simulink model "gm_cruise_control_dut_harness_mq"  (R2014b)
settings: Solver=FixedStepDiscrete  StartTime=0  StopTime=0.029999999999999999  FixedStep=0.01  RelTol=1e-3
undefined symbols (not defined in the file): sigbuilder_block
libraries: simulink x3, hdlmdlgenlib x1, modelsimlib x1
settings Model: RecordCoverage=on  CovMetricSettings=dcmoeb  covSaveCumulativeToWorkspaceVar=off  CovSaveSingleToWorkspaceVar=off  CovReportOnPause=off  CovModelRefEnable=off  CovExternalEMLEnable=on  Creator=The MathWorks Inc.  LastModifiedBy=kotsuka
settings DataIOCC: SaveFormat=StructureWithTime
settings OptimizationCC: BlockReduction=off  ConditionallyExecuteInputs=off  InlineParams=on  InlineInvariantSignals=on  ExpressionFolding=off  ExpressionDepthLimit=2147483647  InitFltsAndDblsToZero=on  EfficientMapNaN2IntZero=off
settings DebuggingCC: SaveWithParameterizedLinksMsg=none  UnderspecifiedInitializationDetection=Classic  MergeDetectMultiDrivingBlocksExec=none  SignalResolutionControl=TryResolveAllWithWarning  InheritedTsInSrcMsg=none  FcnCallInpInsideContextMsg=UseLocalSettings  StateNameClashWarn=warning
settings GRTTargetCC: TargetFcnLib=ansi_tfl_tmw.mat  CombineOutputUpdateFcns=off  GRTInterface=on
settings ConfigComp: Description=Design Verifier Custom Configuration Component  DVMaxProcessTime=60  DVMakeOutputFilesUnique=off  DVParameters=on  DVModelCoverageObjectives=MCDC  DVMaxTestCaseSteps=500  DVTestSuiteOptimization=CombinedObjectives  DVAssertions=EnableAll  DVProofAssumptions=EnableAll  DVCovFilter=on  DVDetectActiveLogic=on  DVProvingStrategy=FindViolation

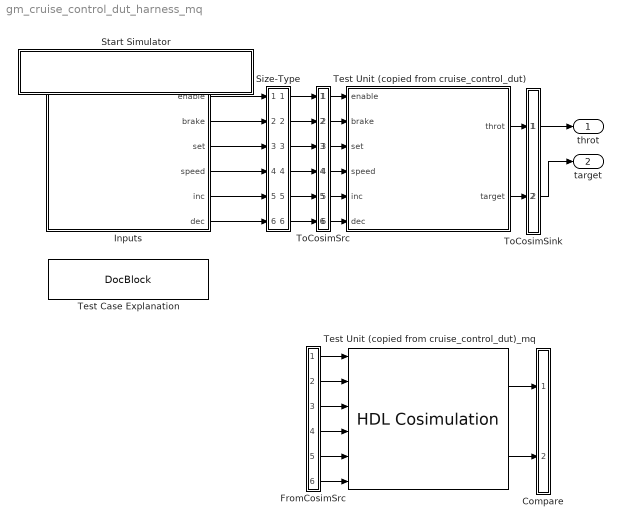
== system gm_cruise_control_dut_harness_mq ==
  Compare : Subsystem
      mask Display: disp('')
  FromCosimSrc : Subsystem
      mask Display: disp('')
  Inputs : Subsystem  Tag=STV Subsys  LoadFcn=sigbuilder_block('load');  StartFcn=sigbuilder_block('start');  StopFcn=sigbuilder_block('stop');  ClipboardFcn=sigbuilder_block('clipboard');  mask(Sigbuilder block){}
      mask init:
      | if ~strcmp(get_param(bdroot(gcb),'SimulationStatus'),'stopped'),tuvar = sigbuilder_block('maskInit'); end
      settings: CopyFcn=sigbuilder_block('copy');  DeleteFcn=sigbuilder_block('delete');  ModelCloseFcn=sigbuilder_block('modelClose');  PreSaveFcn=sigbuilder_block('preSave');  PauseFcn=sigbuilder_block('pause');  ContinueFcn=sigbuilder_block('continue');  NameChangeFcn=sigbuilder_block('namechange');  OpenFcn=sigbuilder_block('open');  CloseFcn=sigbuilder_block('close');
      mask Display: plot(0, 0, 100, 100,[2, 2, 32, 32, 2], [68, 8, 8, 68, 68],[32, 2], [38, 38], [32, 19, 2],[53, 60, 44], [32, 17, 17, 2],[16, 16, 31, 31]);txt = getActiveGroup(gcbh);text(2, 100, txt,'verticalAlignment', 'top');
  Size-Type : Subsystem
  Start Simulator : Subsystem
      settings: OpenFcn=|
      | try
      |    cosimDirName = pwd;
      |    cd 'hdlsrc\cruise_control_dut_harness';
      |    vsim('tclstart',gm_cruise_control_dut_harness_mq_tcl);
      |    cd (cosimDirName);
      |    clear cosimDirName;
      | catch me
      |    disp('Failed to launch cosimulator with "vsim"');
      |    disp (me.message);
      |    cd (cosimDirName);
      |    clear cosimDirName;
      | end
      mask Display: disp(['vsimulink -novopt work.Test_Unit_copied_from_cruise_control_dut' char(10) 'Double-click here to launch ModelSim'])
  Test Case Explanation : simulink/Model-Wide Utilities/DocBlock  DocumentType=Text
  Test Unit (copied from cruise_control_dut) : Subsystem
  Test Unit (copied from cruise_control_dut)_mq : modelsimlib/HDL Cosimulation  PortPaths=/Test_Unit_copied_from_cruise_control_dut/enable;/Test_Unit_copied_from_cruise_control_dut/brake;/Test_Unit_copied_from_cruise_control_dut/set;/Test_Unit_copied_from_cruise_control_dut/speed;/Test_Unit_copied_from_cruise_control_dut/inc;/Test_Unit_copied_from_cruise_control_dut/dec;/Test_Unit_copied_from_cruise_control_dut/throt;/Test_Unit_copied_from_cruise_control_dut/target  PortModes=[1 1 1 1 1 1 2 2 ]  PortTimes=[-1 -1 -1 -1 -1 -1 0.01 0.01 ]  PortSigns=[-1 -1 -1 -1 -1 -1 2 2 ]  PortFracLengths=[0,0,0,0,0,0,0,0]  CommLocal=on  CommSharedMemory=on  CommPortNumber=4449  CommShowInfo=on  ClockModes=[]  ClockTimes=[]  TclPreSimCommand=|  TclPostSimCommand="puts \"done\""  TimingMode=ns  TimingScaleFactor=1000  idxCellArray={'UNUSED_VAR'}  CosimBypass=Full Simulation  AllowDirectFeedthrough=on  ProductName=EDA Simulator Link MQ  RunAutoTimescale=off  HdlClocks=0  PreRunTime=40  PreRunTimeUnit=ns
      | puts "Running Simulink Cosimulation block.";
      |  puts "Chip Name: --> cruise_control_dut_harness/Test Unit (copied from cruise_control_dut)";
      |  puts "Target language: --> vhdl";
      |  puts "Target directory: --> hdlsrc\cruise_control_dut_harness";
      |  puts [clock format [clock seconds]];
      | # Clock force command;
      | force /Test_Unit_copied_from_cruise_control_dut/clk 0 0ns, 1 5ns -r 10ns;
      | # Clock enable force command;
      | force /Test_Unit_copied_from_cruise_control_dut/clk_enable 0 0ns, 1 37ns;
      | # Reset force command;
      | force /Test_Unit_copied_from_cruise_control_dut/reset 1 0ns, 0 27ns;
  ToCosimSink : Subsystem
      mask Display: disp('')
  ToCosimSrc : Subsystem
      mask Display: disp('')
  throt : Outport
  target : Outport  Port=2
  wires:
  Inputs/1(enable) -> Size-Type/1(In1)
  Inputs/2(brake) -> Size-Type/2(In2)
  Inputs/3(set) -> Size-Type/3(In3)
  Inputs/4(speed) -> Size-Type/4(In4)
  Inputs/5(inc) -> Size-Type/5(In5)
  Inputs/6(dec) -> Size-Type/6(In6)
  ToCosimSrc/1(out1) -> Test Unit (copied from cruise_control_dut)/1(enable)
  ToCosimSrc/2(out2) -> Test Unit (copied from cruise_control_dut)/2(brake)
  ToCosimSrc/3(out3) -> Test Unit (copied from cruise_control_dut)/3(set)
  ToCosimSrc/4(out4) -> Test Unit (copied from cruise_control_dut)/4(speed)
  ToCosimSrc/5(out5) -> Test Unit (copied from cruise_control_dut)/5(inc)
  ToCosimSrc/6(out6) -> Test Unit (copied from cruise_control_dut)/6(dec)
  Test Unit (copied from cruise_control_dut)/1(throt) -> ToCosimSink/1(in1)
  Test Unit (copied from cruise_control_dut)/2(target) -> ToCosimSink/2(in2)
  Size-Type/1(Out1) -> ToCosimSrc/1(in1)
  Size-Type/2(Out2) -> ToCosimSrc/2(in2)
  Size-Type/3(Out3) -> ToCosimSrc/3(in3)
  Size-Type/4(Out4) -> ToCosimSrc/4(in4)
  Size-Type/5(Out5) -> ToCosimSrc/5(in5)
  Size-Type/6(Out6) -> ToCosimSrc/6(in6)
  ToCosimSink/1(out1) -> throt/1
  ToCosimSink/2(out2) -> target/1
  FromCosimSrc/1(out1) -> Test Unit (copied from cruise_control_dut)_mq/1
  FromCosimSrc/2(out2) -> Test Unit (copied from cruise_control_dut)_mq/2
  FromCosimSrc/3(out3) -> Test Unit (copied from cruise_control_dut)_mq/3
  FromCosimSrc/4(out4) -> Test Unit (copied from cruise_control_dut)_mq/4
  FromCosimSrc/5(out5) -> Test Unit (copied from cruise_control_dut)_mq/5
  FromCosimSrc/6(out6) -> Test Unit (copied from cruise_control_dut)_mq/6
  Test Unit (copied from cruise_control_dut)_mq/1 -> Compare/1(in1)
  Test Unit (copied from cruise_control_dut)_mq/2 -> Compare/2(in2)

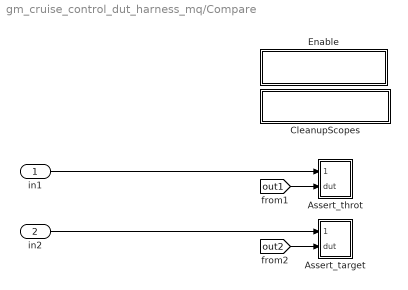
== system gm_cruise_control_dut_harness_mq/Compare ==
  in1 : Inport
  in2 : Inport  Port=2
  Assert_target : Subsystem
  Assert_throt : Subsystem
  CleanupScopes : Subsystem
      settings: OpenFcn=|
      | blkName = gcb;
      | idx = regexp(blkName, '/CleanupScopes$', 'once');
      | blkParent = blkName(1:idx-1);
      | blks=find_system(blkParent, 'blocktype', 'Scope');
      | e = get_param(blks{1}, 'Open');
      | if strcmp(e, 'on'), f= 'off'; else f = 'on'; end
      | for ii=1:length(blks), set_param(blks{ii}, 'Open', f); end; drawnow;
      mask Display: disp(['Double click to\n turn on/off all scopes'])
  Enable : Subsystem
      settings: OpenFcn=|
      | blkName = gcb;
      | idx = regexp(blkName, '/Enable$', 'once');
      | blkParent = blkName(1:idx-1);
      | blks=find_system(blkParent, 'blocktype', 'Assertion');
      | e = get_param(blks{1}, 'Enabled');
      | if strcmp(e, 'on'), f= 'off';, else, f = 'on';, end
      | for ii=1:length(blks), set_param(blks{ii}, 'Enabled', f);, end
      | dispMsg = sprintf('disp([''Double click to turn %s \\n all Assertions''])', upper(e));
      | set_param(gcb, 'MaskDisplay', dispMsg);
      mask Display: disp(['Double click to turn OFF \n all Assertions'])
  wires:
  in1/1 -> Assert_throt/1(cosim)
  [out1] -> Assert_throt/2(dut)
  in2/1 -> Assert_target/1(cosim)
  [out2] -> Assert_target/2(dut)

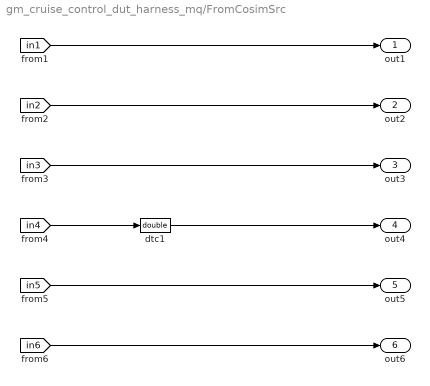
== system gm_cruise_control_dut_harness_mq/FromCosimSrc ==
  dtc1 : DataTypeConversion  OutDataTypeStr=double  SaturateOnIntegerOverflow=on  RndMeth=Zero
  out1 : Outport
  out2 : Outport  Port=2
  out3 : Outport  Port=3
  out4 : Outport  Port=4
  out5 : Outport  Port=5
  out6 : Outport  Port=6
  wires:
  [in4] -> dtc1/1
  [in1] -> out1/1
  [in2] -> out2/1
  [in3] -> out3/1
  dtc1/1 -> out4/1
  [in5] -> out5/1
  [in6] -> out6/1

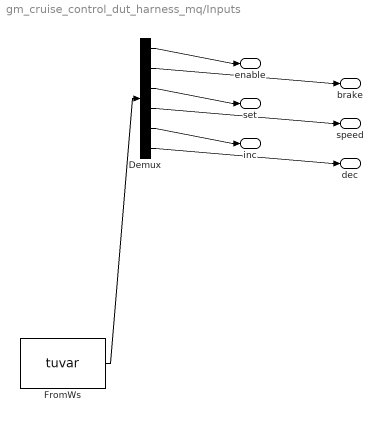
== system gm_cruise_control_dut_harness_mq/Inputs ==
  Demux : Demux  Tag=STV Demux  Outputs=6
  FromWs : FromWorkspace  Tag=STV FromWs  VariableName=tuvar  SampleTime=0
      SigBuilderData=|
      | dataSet(1).timeRange = [0 0.01]
      | dataSet(1).name = 'テスト ケース 1'
      | dataSet(2).timeRange = [0 0.01]
      | dataSet(2).name = 'テスト ケース 2'
      | dataSet(3).timeRange = [0 0.01]
      | dataSet(3).name = 'テスト ケース 3'
      | dataSet(4).timeRange = [0 0.01]
      | dataSet(4).name = 'テスト ケース 4'
      | dataSet(5).timeRange = [0 0.01]
      | dataSet(5).name = 'テスト ケース 5'
      | dataSet(6).timeRange = [0 0.01]
      | dataSet(6).name = 'テスト ケース 6'
      | dataSet(7).timeRange = [0 0.02]
      | dataSet(7).name = 'テスト ケース 7'
      | dataSet(8).timeRange = [0 0.03]
      | dataSet(8).name = 'テスト ケース 8'
      | dataSet(9).timeRange = [0 0.03]
      | dataSet(9).name = 'テスト ケース 9'
      | sbobj.Name = 'Signal Builder'
      | sbobj.Groups(1).Name = 'テスト ケース 1'
      | sbobj.Groups(1).Signals(1).Name = 'enable'
      | sbobj.Groups(1).Signals(1).XData = [0 0.01]
      | sbobj.Groups(1).Signals(1).YData = [0 0]
      | sbobj.Groups(1).Signals(2).Name = 'brake'
      | sbobj.Groups(1).Signals(2).XData = [0 0.01]
      | sbobj.Groups(1).Signals(2).YData = [0 0]
      | sbobj.Groups(1).Signals(3).Name = 'set'
      | sbobj.Groups(1).Signals(3).XData = [0 0.01]
      | sbobj.Groups(1).Signals(3).YData = [1 1]
      | sbobj.Groups(1).Signals(4).Name = 'speed'
      | sbobj.Groups(1).Signals(4).XData = [0 0.01]
      | sbobj.Groups(1).Signals(4).YData = [0 0]
      | sbobj.Groups(1).Signals(5).Name = 'inc'
      | sbobj.Groups(1).Signals(5).XData = [0 0.01]
      | sbobj.Groups(1).Signals(5).YData = [0 0]
      | sbobj.Groups(1).Signals(6).Name = 'dec'
      | sbobj.Groups(1).Signals(6).XData = [0 0.01]
      | sbobj.Groups(1).Signals(6).YData = [0 0]
      | sbobj.Groups(1).TimeRange = [0 0.01]
      | sbobj.Groups(2).Name = 'テスト ケース 2'
      | sbobj.Groups(2).Signals(1).Name = 'enable'
      | sbobj.Groups(2).Signals(1).XData = [0 0.01]
      | sbobj.Groups(2).Signals(1).YData = [1 1]
      | sbobj.Groups(2).Signals(2).Name = 'brake'
      | sbobj.Groups(2).Signals(2).XData = [0 0.01]
      | sbobj.Groups(2).Signals(2).YData = [1 1]
      | sbobj.Groups(2).Signals(3).Name = 'set'
      | sbobj.Groups(2).Signals(3).XData = [0 0.01]
      | sbobj.Groups(2).Signals(3).YData = [1 1]
      | sbobj.Groups(2).Signals(4).Name = 'speed'
      | sbobj.Groups(2).Signals(4).XData = [0 0.01]
      | sbobj.Groups(2).Signals(4).YData = [0 0]
      | sbobj.Groups(2).Signals(5).Name = 'inc'
      | sbobj.Groups(2).Signals(5).XData = [0 0.01]
      | sbobj.Groups(2).Signals(5).YData = [0 0]
      | sbobj.Groups(2).Signals(6).Name = 'dec'
      | sbobj.Groups(2).Signals(6).XData = [0 0.01]
      | sbobj.Groups(2).Signals(6).YData = [0 0]
      | sbobj.Groups(2).TimeRange = [0 0.01]
      | sbobj.Groups(3).Name = 'テスト ケース 3'
      | sbobj.Groups(3).Signals(1).Name = 'enable'
      | sbobj.Groups(3).Signals(1).XData = [0 0.01]
      | sbobj.Groups(3).Signals(1).YData = [0 0]
      | sbobj.Groups(3).Signals(2).Name = 'brake'
      | sbobj.Groups(3).Signals(2).XData = [0 0.01]
      | sbobj.Groups(3).Signals(2).YData = [0 0]
      | sbobj.Groups(3).Signals(3).Name = 'set'
      | sbobj.Groups(3).Signals(3).XData = [0 0.01]
      | sbobj.Groups(3).Signals(3).YData = [0 0]
      | sbobj.Groups(3).Signals(4).Name = 'speed'
      | sbobj.Groups(3).Signals(4).XData = [0 0.01]
      | sbobj.Groups(3).Signals(4).YData = [0 0]
      | sbobj.Groups(3).Signals(5).Name = 'inc'
      | sbobj.Groups(3).Signals(5).XData = [0 0.01]
      | sbobj.Groups(3).Signals(5).YData = [1 1]
      | sbobj.Groups(3).Signals(6).Name = 'dec'
      | sbobj.Groups(3).Signals(6).XData = [0 0.01]
      | sbobj.Groups(3).Signals(6).YData = [0 0]
      | sbobj.Groups(3).TimeRange = [0 0.01]
      | sbobj.Groups(4).Name = 'テスト ケース 4'
      | sbobj.Groups(4).Signals(1).Name = 'enable'
      | sbobj.Groups(4).Signals(1).XData = [0 0.01]
      | sbobj.Groups(4).Signals(1).YData = [1 1]
      | sbobj.Groups(4).Signals(2).Name = 'brake'
      | sbobj.Groups(4).Signals(2).XData = [0 0.01]
      | sbobj.Groups(4).Signals(2).YData = [0 0]
      | sbobj.Groups(4).Signals(3).Name = 'set'
      | sbobj.Groups(4).Signals(3).XData = [0 0.01]
      | sbobj.Groups(4).Signals(3).YData = [0 0]
      | sbobj.Groups(4).Signals(4).Name = 'speed'
      | sbobj.Groups(4).Signals(4).XData = [0 0.01]
      | sbobj.Groups(4).Signals(4).YData = [0 0]
      | sbobj.Groups(4).Signals(5).Name = 'inc'
      | sbobj.Groups(4).Signals(5).XData = [0 0.01]
      | sbobj.Groups(4).Signals(5).YData = [1 1]
      | sbobj.Groups(4).Signals(6).Name = 'dec'
      | sbobj.Groups(4).Signals(6).XData = [0 0.01]
      | sbobj.Groups(4).Signals(6).YData = [0 0]
      | sbobj.Groups(4).TimeRange = [0 0.01]
      | sbobj.Groups(5).Name = 'テスト ケース 5'
      | sbobj.Groups(5).Signals(1).Name = 'enable'
      | sbobj.Groups(5).Signals(1).XData = [0 0.01]
      | sbobj.Groups(5).Signals(1).YData = [1 1]
      | sbobj.Groups(5).Signals(2).Name = 'brake'
      | sbobj.Groups(5).Signals(2).XData = [0 0.01]
      | sbobj.Groups(5).Signals(2).YData = [0 0]
      | sbobj.Groups(5).Signals(3).Name = 'set'
      | sbobj.Groups(5).Signals(3).XData = [0 0.01]
      | sbobj.Groups(5).Signals(3).YData = [1 1]
      | sbobj.Groups(5).Signals(4).Name = 'speed'
      | sbobj.Groups(5).Signals(4).XData = [0 0.01]
      | sbobj.Groups(5).Signals(4).YData = [0 0]
      | sbobj.Groups(5).Signals(5).Name = 'inc'
      | sbobj.Groups(5).Signals(5).XData = [0 0.01]
      | sbobj.Groups(5).Signals(5).YData = [0 0]
      | sbobj.Groups(5).Signals(6).Name = 'dec'
      | sbobj.Groups(5).Signals(6).XData = [0 0.01]
      | sbobj.Groups(5).Signals(6).YData = [0 0]
      | sbobj.Groups(5).TimeRange = [0 0.01]
      | sbobj.Groups(6).Name = 'テスト ケース 6'
      | sbobj.Groups(6).Signals(1).Name = 'enable'
      | sbobj.Groups(6).Signals(1).XData = [0 0.01]
      | sbobj.Groups(6).Signals(1).YData = [0 0]
      | sbobj.Groups(6).Signals(2).Name = 'brake'
      | sbobj.Groups(6).Signals(2).XData = [0 0.01]
      | sbobj.Groups(6).Signals(2).YData = [0 0]
      | sbobj.Groups(6).Signals(3).Name = 'set'
      | sbobj.Groups(6).Signals(3).XData = [0 0.01]
      | sbobj.Groups(6).Signals(3).YData = [1 1]
      | sbobj.Groups(6).Signals(4).Name = 'speed'
      | sbobj.Groups(6).Signals(4).XData = [0 0.01]
      | sbobj.Groups(6).Signals(4).YData = [0 0]
      | sbobj.Groups(6).Signals(5).Name = 'inc'
      | sbobj.Groups(6).Signals(5).XData = [0 0.01]
      | sbobj.Groups(6).Signals(5).YData = [0 0]
      | sbobj.Groups(6).Signals(6).Name = 'dec'
      | sbobj.Groups(6).Signals(6).XData = [0 0.01]
      | sbobj.Groups(6).Signals(6).YData = [1 1]
      | sbobj.Groups(6).TimeRange = [0 0.01]
      | sbobj.Groups(7).Name = 'テスト ケース 7'
      | sbobj.Groups(7).Signals(1).Name = 'enable'
      | sbobj.Groups(7).Signals(1).XData = [0 0.01 0.02]
      | sbobj.Groups(7).Signals(1).YData = [1 1 1]
      | sbobj.Groups(7).Signals(2).Name = 'brake'
      | sbobj.Groups(7).Signals(2).XData = [0 0.01 0.02]
      | sbobj.Groups(7).Signals(2).YData = [0 0 0]
      | sbobj.Groups(7).Signals(3).Name = 'set'
      | sbobj.Groups(7).Signals(3).XData = [0 0.01 0.01 0.02]
      | sbobj.Groups(7).Signals(3).YData = [1 1 0 0]
      | sbobj.Groups(7).Signals(4).Name = 'speed'
      | sbobj.Groups(7).Signals(4).XData = [0 0.01 0.02]
      | sbobj.Groups(7).Signals(4).YData = [0 0 0]
      | sbobj.Groups(7).Signals(5).Name = 'inc'
      | sbobj.Groups(7).Signals(5).XData = [0 0.01 0.01 0.02]
      | sbobj.Groups(7).Signals(5).YData = [1 1 0 0]
      | sbobj.Groups(7).Signals(6).Name = 'dec'
      | sbobj.Groups(7).Signals(6).XData = [0 0.01 0.02]
      | sbobj.Groups(7).Signals(6).YData = [0 0 0]
      | sbobj.Groups(7).TimeRange = [0 0.02]
      | sbobj.Groups(8).Name = 'テスト ケース 8'
      | sbobj.Groups(8).Signals(1).Name = 'enable'
      | sbobj.Groups(8).Signals(1).XData = [0 0.01 0.02 0.03]
      | sbobj.Groups(8).Signals(1).YData = [1 1 1 1]
      | sbobj.Groups(8).Signals(2).Name = 'brake'
      | sbobj.Groups(8).Signals(2).XData = [0 0.01 0.02 0.03]
      | sbobj.Groups(8).Signals(2).YData = [0 0 0 0]
      | sbobj.Groups(8).Signals(3).Name = 'set'
      | sbobj.Groups(8).Signals(3).XData = [0 0.01 0.01 0.02 0.02 0.03]
      | sbobj.Groups(8).Signals(3).YData = [1 1 0 0 1 1]
      | sbobj.Groups(8).Signals(4).Name = 'speed'
      | sbobj.Groups(8).Signals(4).XData = [0 0.01 0.01 0.02 0.02 0.03]
      | sbobj.Groups(8).Signals(4).YData = [0 0 -499 -499 0 0]
      | sbobj.Groups(8).Signals(5).Name = 'inc'
      | sbobj.Groups(8).Signals(5).XData = [0 0.01 0.02 0.02 0.03]
      | sbobj.Groups(8).Signals(5).YData = [1 1 1 0 0]
      | sbobj.Groups(8).Signals(6).Name = 'dec'
      | sbobj.Groups(8).Signals(6).XData = [0 0.01 0.02 0.03]
      | sbobj.Groups(8).Signals(6).YData = [0 0 0 0]
      | sbobj.Groups(8).TimeRange = [0 0.03]
      | sbobj.Groups(9).Name = 'テスト ケース 9'
      | sbobj.Groups(9).Signals(1).Name = 'enable'
      | sbobj.Groups(9).Signals(1).XData = [0 0.01 0.02 0.03]
      | sbobj.Groups(9).Signals(1).YData = [1 1 1 1]
      | sbobj.Groups(9).Signals(2).Name = 'brake'
      | sbobj.Groups(9).Signals(2).XData = [0 0.01 0.02 0.03]
      | sbobj.Groups(9).Signals(2).YData = [0 0 0 0]
      | sbobj.Groups(9).Signals(3).Name = 'set'
      | sbobj.Groups(9).Signals(3).XData = [0 0.01 0.01 0.02 0.02 0.03]
      | sbobj.Groups(9).Signals(3).YData = [1 1 0 0 1 1]
      | sbobj.Groups(9).Signals(4).Name = 'speed'
      | sbobj.Groups(9).Signals(4).XData = [0 0.01 0.01 0.02 0.02 0.03]
      | sbobj.Groups(9).Signals(4).YData = [0 0 501 501 0 0]
      | sbobj.Groups(9).Signals(5).Name = 'inc'
      | sbobj.Groups(9).Signals(5).XData = [0 0.01 0.02 0.02 0.03]
      | sbobj.Groups(9).Signals(5).YData = [1 1 1 0 0]
      | sbobj.Groups(9).Signals(6).Name = 'dec'
      | sbobj.Groups(9).Signals(6).XData = [0 0.01 0.02 0.03]
      | sbobj.Groups(9).Signals(6).YData = [0 0 0 0]
      | sbobj.Groups(9).TimeRange = [0 0.03]
  enable : Outport  Tag=STV Outport
  brake : Outport  Tag=STV Outport  Port=2
  set : Outport  Tag=STV Outport  Port=3
  speed : Outport  Tag=STV Outport  Port=4
  inc : Outport  Tag=STV Outport  Port=5
  dec : Outport  Tag=STV Outport  Port=6
  wires:
  FromWs/1 -> Demux/1
  Demux/1 -> enable/1
  Demux/2 -> brake/1
  Demux/3 -> set/1
  Demux/4 -> speed/1
  Demux/5 -> inc/1
  Demux/6 -> dec/1

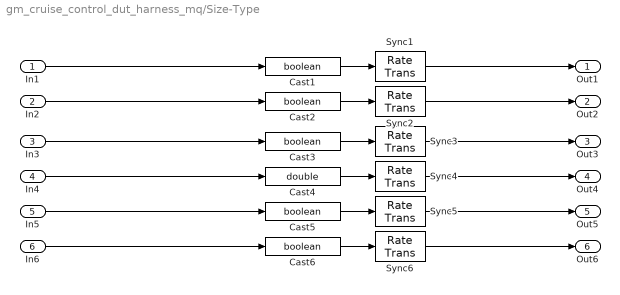
== system gm_cruise_control_dut_harness_mq/Size-Type ==
  In1 : Inport
  In2 : Inport  Port=2
  In3 : Inport  Port=3
  In4 : Inport  Port=4
  In5 : Inport  Port=5
  In6 : Inport  Port=6
  Cast{1..3,5..6} (5 alike) : DataTypeConversion  OutDataTypeStr=boolean  RndMeth=Nearest  SaturateOnIntegerOverflow=on
  Cast4 : DataTypeConversion  OutDataTypeStr=double  RndMeth=Nearest  SaturateOnIntegerOverflow=on
  Sync{1..6} (6 alike) : RateTransition  OutPortSampleTime=[0.01,0]
  Out1 : Outport
  Out2 : Outport  Port=2
  Out3 : Outport  Port=3
  Out4 : Outport  Port=4
  Out5 : Outport  Port=5
  Out6 : Outport  Port=6
  wires:
  In1/1 -> Cast1/1
  Cast1/1 -> Sync1/1
  Sync1/1 -> Out1/1
  In2/1 -> Cast2/1
  Cast2/1 -> Sync2/1
  Sync2/1 -> Out2/1
  In3/1 -> Cast3/1
  Cast3/1 -> Sync3/1
  Sync3/1 -> Out3/1
  In4/1 -> Cast4/1
  Cast4/1 -> Sync4/1
  Sync4/1 -> Out4/1
  In5/1 -> Cast5/1
  Cast5/1 -> Sync5/1
  Sync5/1 -> Out5/1
  In6/1 -> Cast6/1
  Cast6/1 -> Sync6/1
  Sync6/1 -> Out6/1

== system gm_cruise_control_dut_harness_mq/Start Simulator ==

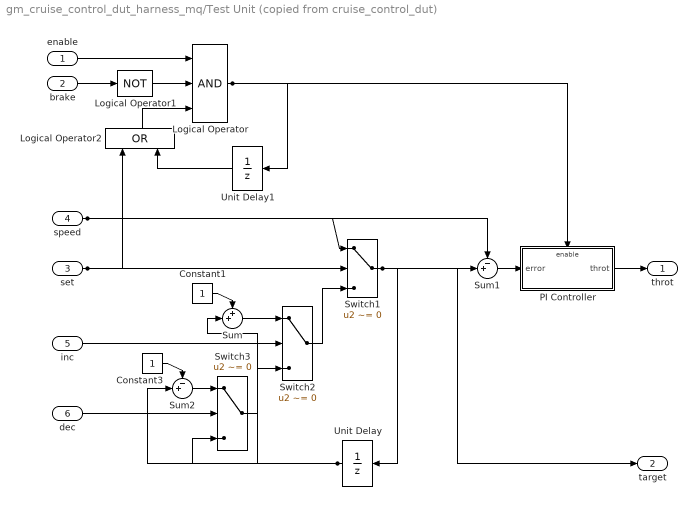
== system gm_cruise_control_dut_harness_mq/Test Unit (copied from cruise_control_dut) ==
  enable : Inport  OutDataTypeStr=boolean
  brake : Inport  Port=2  OutDataTypeStr=boolean
  set : Inport  Port=3  OutDataTypeStr=boolean
  speed : Inport  Port=4  OutDataTypeStr=double
  inc : Inport  Port=5  OutDataTypeStr=boolean
  dec : Inport  Port=6  OutDataTypeStr=boolean
  Constant1 : Constant
  Constant3 : Constant
  Logical Operator : Logic  Inputs=3  AllPortsSameDT=off  OutDataTypeStr=boolean
  Logical Operator1 : Logic  Operator=NOT  AllPortsSameDT=off  OutDataTypeStr=boolean
  Logical Operator2 : Logic  Operator=OR  AllPortsSameDT=off  OutDataTypeStr=boolean
  PI Controller : Subsystem
  Sum : Sum  Inputs=++|
  Sum1 : Sum  Inputs=-+|
  Sum2 : Sum  Inputs=-+|
  Switch1 : Switch  Criteria=u2 ~= 0
  Switch2 : Switch  Criteria=u2 ~= 0
  Switch3 : Switch  Criteria=u2 ~= 0
  Unit Delay : UnitDelay  SampleTime=0.01
  Unit Delay1 : UnitDelay  SampleTime=0.01
  throt : Outport
  target : Outport  Port=2
  wires:
  Unit Delay1/1 -> Logical Operator2/2
  Unit Delay/1 -> Sum/2, Sum2/2, Switch3/3
  Switch3/1 -> Switch2/3
  Switch2/1 -> Switch1/3
  Switch1/1 -> target/1, Unit Delay/1, Sum1/2
  Sum2/1 -> Switch3/1
  Sum1/1 -> PI Controller/1(error)
  Sum/1 -> Switch2/1
  PI Controller/1(throt) -> throt/1
  Logical Operator2/1 -> Logical Operator/3
  Logical Operator1/1 -> Logical Operator/2
  Logical Operator/1 -> PI Controller/Enable, Unit Delay1/1
  Constant3/1 -> Sum2/1
  Constant1/1 -> Sum/1
  dec/1 -> Switch3/2
  inc/1 -> Switch2/2
  speed/1 -> Sum1/1, Switch1/1
  set/1 -> Logical Operator2/1, Switch1/2
  brake/1 -> Logical Operator1/1
  enable/1 -> Logical Operator/1

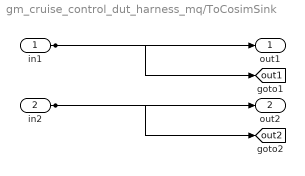
== system gm_cruise_control_dut_harness_mq/ToCosimSink ==
  in1 : Inport
  in2 : Inport  Port=2
  out1 : Outport
  out2 : Outport  Port=2
  tag scope: out1=global, out2=global
  wires:
  in1/1 -> out1/1, [out1]
  in2/1 -> out2/1, [out2]

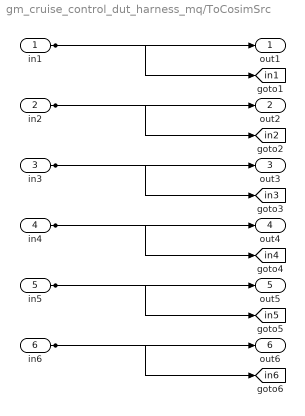
== system gm_cruise_control_dut_harness_mq/ToCosimSrc ==
  in1 : Inport
  in2 : Inport  Port=2
  in3 : Inport  Port=3
  in4 : Inport  Port=4
  in5 : Inport  Port=5
  in6 : Inport  Port=6
  out1 : Outport
  out2 : Outport  Port=2
  out3 : Outport  Port=3
  out4 : Outport  Port=4
  out5 : Outport  Port=5
  out6 : Outport  Port=6
  tag scope: in1=global, in2=global, in3=global, in4=global, in5=global, in6=global
  wires:
  in1/1 -> out1/1, [in1]
  in2/1 -> out2/1, [in2]
  in3/1 -> out3/1, [in3]
  in4/1 -> out4/1, [in4]
  in5/1 -> out5/1, [in5]
  in6/1 -> out6/1, [in6]

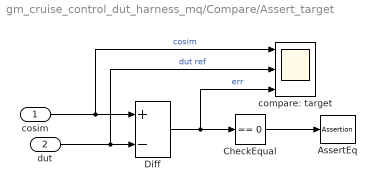
== system gm_cruise_control_dut_harness_mq/Compare/Assert_target ==
  cosim : Inport
  dut : Inport  Port=2
  AssertEq : Assertion  StopWhenAssertionFail=off
  CheckEqual : simulink/Logic and Bit Operations/Compare To Zero  relop===  OutDataTypeStr=uint8  ZeroCross=off
  Diff : Sum  Inputs=+-
  compare: target : Scope  NumInputPorts=3
      settings: YMin=-5~-5~-5  YMax=5~5~5
  wires:
  CheckEqual/1 -> AssertEq/1
  dut/1 -> Diff/2, compare: target/2  "dut ref"
  cosim/1 -> compare: target/1, Diff/1  "cosim"
  Diff/1 -> CheckEqual/1, compare: target/3  "err"

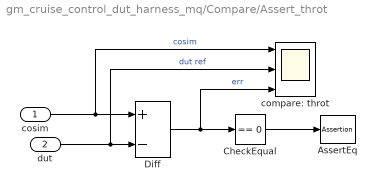
== system gm_cruise_control_dut_harness_mq/Compare/Assert_throt ==
  cosim : Inport
  dut : Inport  Port=2
  AssertEq : Assertion  StopWhenAssertionFail=off
  CheckEqual : simulink/Logic and Bit Operations/Compare To Zero  relop===  OutDataTypeStr=uint8  ZeroCross=off
  Diff : Sum  Inputs=+-
  compare: throt : Scope  NumInputPorts=3
      settings: YMin=-5~-5~-5  YMax=5~5~5
  wires:
  CheckEqual/1 -> AssertEq/1
  dut/1 -> Diff/2, compare: throt/2  "dut ref"
  cosim/1 -> compare: throt/1, Diff/1  "cosim"
  Diff/1 -> CheckEqual/1, compare: throt/3  "err"

== system gm_cruise_control_dut_harness_mq/Compare/CleanupScopes ==

== system gm_cruise_control_dut_harness_mq/Compare/Enable ==

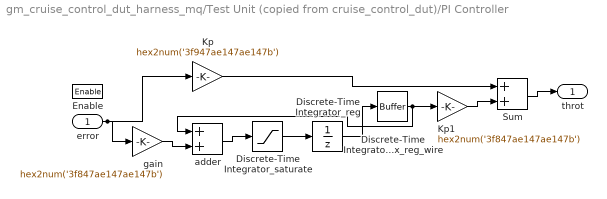
== system gm_cruise_control_dut_harness_mq/Test Unit (copied from cruise_control_dut)/PI Controller ==
  error : Inport
  Enable : EnablePort
  Discrete-Time Integrator_reg : UnitDelay  InitialCondition=hex2num('0000000000000000')  SampleTime=0.01
  Discrete-Time Integrator_saturate : Saturate  UpperLimit=hex2num('4014000000000000')  LowerLimit=hex2num('c014000000000000')  SampleTime=0.01  OutDataTypeStr=double
  Discrete-Time Integrator_x_reg_wire : hdlmdlgenlib/Buffer
  Kp : Gain  Gain=hex2num('3f947ae147ae147b')  OutDataTypeStr=double  SampleTime=0.01
  Kp1 : Gain  Gain=hex2num('3f847ae147ae147b')  OutDataTypeStr=double  SampleTime=0.01
  Sum : Sum  AccumDataTypeStr=double  OutDataTypeStr=double  SampleTime=0.01
  adder : Sum  AccumDataTypeStr=double  OutDataTypeStr=double  SampleTime=0.01
  gain : Gain  Gain=hex2num('3f847ae147ae147b')  OutDataTypeStr=double  SampleTime=0.01
  throt : Outport  InitialOutput=0
  wires:
  Discrete-Time Integrator_reg/1 -> Discrete-Time Integrator_x_reg_wire/1
  Discrete-Time Integrator_saturate/1 -> Discrete-Time Integrator_reg/1
  adder/1 -> Discrete-Time Integrator_saturate/1
  gain/1 -> adder/2
  Sum/1 -> throt/1
  Kp1/1 -> Sum/2
  Kp/1 -> Sum/1
  Discrete-Time Integrator_x_reg_wire/1 -> adder/1, Kp1/1
  error/1 -> gain/1, Kp/1
